simulink model "child"  (R2023a)
settings: Solver=FixedStepDiscrete  StartTime=0.0  StopTime=inf  RelTol=1e-3
undefined symbols (not defined in the file): child_1, dismiss
libraries: androidcommunicationlib x9, androidaudiovideolib x3, androidsensorlib x3, simulink x2, androiduilib x1
settings Model: SimulationMode=external  Creator=aashm  LastModifiedBy=agarw_crynhxp
settings OptimizationCC: BlockReduction=off  EnhancedBackFolding=on  PassReuseOutputArgsAs=Individual arguments  ZeroExternalMemoryAtStartup=off  ZeroInternalMemoryAtStartup=off  MaxStackSize=64  OptimizeBlockOrder=speed  DifferentSizesBufferReuse=on  OptimizationCustomize=off  EfficientTunableParamExpr=on
settings DebuggingCC: ParameterTunabilityLossMsg=error
settings HardwareCC: ProdBitPerPointer=32  ProdBitPerSizeT=32  ProdBitPerPtrDiffT=32  ProdLargestAtomicInteger=Long  ProdLargestAtomicFloat=Double  ProdWordSize=32  ProdHWDeviceType=ARM Compatible->ARM Cortex  UseEmbeddedCoderFeatures=off  UseSimulinkCoderFeatures=off
settings SFSimCC: MATLABDynamicMemAlloc=off
settings RTWCC: Description=Embedded Coder  SystemTargetFile=ert.tlc  HardwareBoard=Android Device  TLCOptions="-aInlineSetEventsForThisBaseRateFcn=TLC_FALSE -aSuppressMultiTaskScheduler=TLC_FALSE  -aRateBasedStepFcn=0"  TemplateMakefile=ert_default_tmf  RTWVerbose=off  Toolchain=Android SDK/NDK Tools
settings CodeAppCC: ForceParamTrailComments=on  IgnoreCustomStorageClasses=off  OperatorAnnotations=on  SimulinkDataObjDesc=on  SFDataObjDesc=on  InsertBlockDesc=on
settings ERTTargetCC: SupportNonInlinedSFcns=on

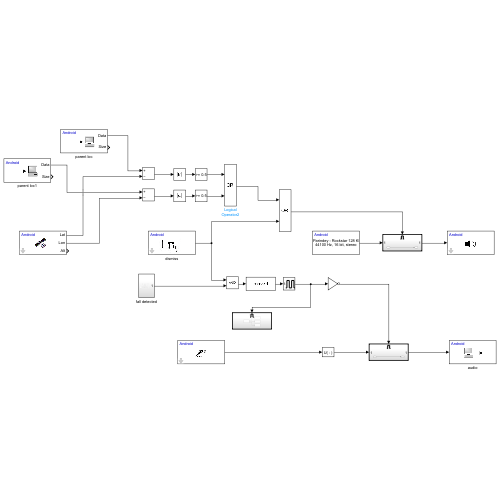
[thumbnail: Simulink's stored preview of the top-level diagram]
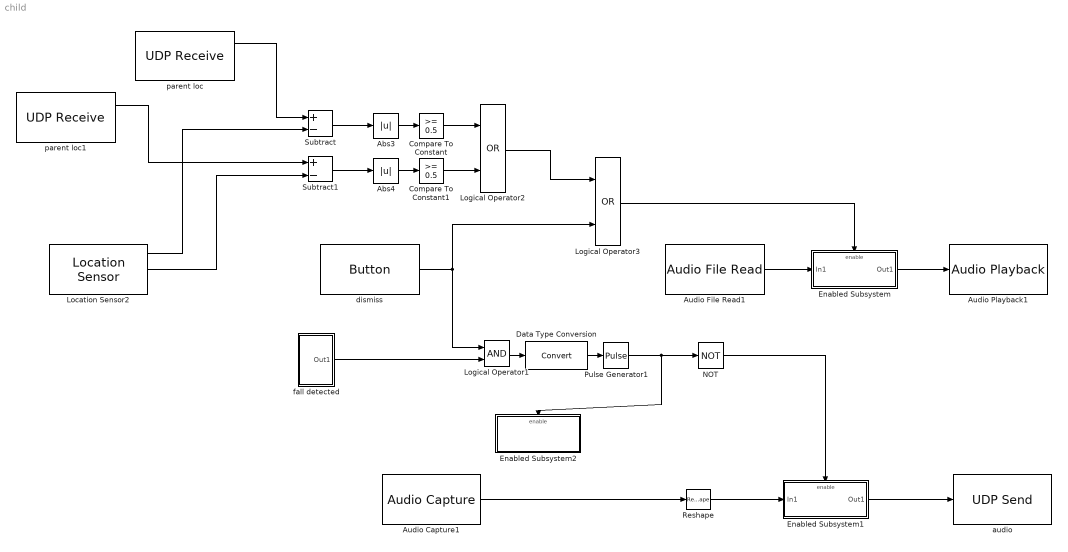
== system child ==
  Abs3 : Abs  OutDataTypeStr=int8  SaturateOnIntegerOverflow=off
  Abs4 : Abs  OutDataTypeStr=int8  SaturateOnIntegerOverflow=off
  Audio Capture1 : androidaudiovideolib/Audio Capture  SampleFreq=8000  FrameSize=80  SampleTime=0.01  SimulateUsing=Code generation  DeviceStr=0  QueueDuration=0  BlockPlatform=Android  AudioSamplingFreq=44100
  Audio File Read1 : androidaudiovideolib/Audio File Read  FileName=E:\agarw_crynhxp\Documents\Nadaan Parindey - Rockstar 128 Kbps.mp3  FrameSize=44100
  Audio Playback1 : androidaudiovideolib/Audio Playback  SampleFreq=44100  AudioSamplingFreq=44100  SampleTime=0.1  DeviceStr=0  QueueDuration=0  BlockPlatform=Android
  Compare To Constant : simulink/Logic and Bit Operations/Compare To Constant  relop=>=  const=0.5  OutDataTypeStr=boolean
  Compare To Constant1 : simulink/Logic and Bit Operations/Compare To Constant  relop=>=  const=0.5  OutDataTypeStr=boolean
  Data Type Conversion : DataTypeConversion  SaturateOnIntegerOverflow=off  RndMeth=Floor
  Enabled Subsystem : Subsystem  TreatAsAtomicUnit=on
  Enabled Subsystem1 : Subsystem  TreatAsAtomicUnit=on
  Enabled Subsystem2 : Subsystem  TreatAsAtomicUnit=on
  Location Sensor2 : androidsensorlib/Location Sensor  OutputVector=off  SampleTime=0.01  BlockPlatform=Android
  Logical Operator1 : Logic  AllPortsSameDT=off  OutDataTypeStr=fixdt(1,16)
  Logical Operator2 : Logic  Operator=OR  OutDataTypeStr=boolean
  Logical Operator3 : Logic  Operator=OR
  NOT : Logic  Operator=NOT  IconShape=distinctive  AllPortsSameDT=off
  Pulse Generator1 : DiscretePulseGenerator  PulseType=Time based  TimeSource=Use external signal  Period=100  PulseWidth=5
  Reshape : Reshape
  Subtract : Sum  Inputs=+-  OutDataTypeStr=int8
  Subtract1 : Sum  Inputs=+-  AccumDataTypeStr=int8  OutDataTypeStr=int8
  audio : androidcommunicationlib/UDP Send  remoteURL='10.7.20.4'  remotePort=30000  localURL='0.0.0.0'  localPortSource=Automatically determine  localPort=-1  sampletime=-1  blockPlatform=Android  separateLengthPort=0
  dismiss : androiduilib/Button  ButtonState=Pressed  ButtonId=child_1/dismiss  State=on  SampleTime=0.1  BlockPlatform=Android
  fall detected : Subsystem
  parent loc : androidcommunicationlib/UDP Receive  localURL='0.0.0.0'  localPort=40000  remoteURL='0.0.0.0'  remotePort=-1  recvBufferSize=8192  signalDatatype=uint8  dims=255  isVarSize=off  showBlockingTime=off  blockingTime=0  sampletime=0.01  blockPlatform=Android
  parent loc1 : androidcommunicationlib/UDP Receive  localURL='0.0.0.0'  localPort=45000  remoteURL='0.0.0.0'  remotePort=-1  recvBufferSize=8192  signalDatatype=uint8  dims=255  isVarSize=off  showBlockingTime=off  blockingTime=0  sampletime=0.01  blockPlatform=Android
  wires:
  dismiss/1 -> Logical Operator1/1, Logical Operator3/2
  Pulse Generator1/1 -> Enabled Subsystem2/Enable, NOT/1
  Enabled Subsystem1/1(Out1) -> audio/1
  Subtract/1 -> Abs3/1
  Compare To Constant/1 -> Logical Operator2/1
  Abs3/1 -> Compare To Constant/1
  Location Sensor2/1 -> Subtract/2
  Subtract1/1 -> Abs4/1
  Abs4/1 -> Compare To Constant1/1
  parent loc1/1 -> Subtract1/1
  Location Sensor2/2 -> Subtract1/2
  Compare To Constant1/1 -> Logical Operator2/2
  Audio Capture1/1 -> Reshape/1
  Reshape/1 -> Enabled Subsystem1/1(In1)
  Logical Operator2/1 -> Logical Operator3/1
  parent loc/1 -> Subtract/1
  Audio File Read1/1 -> Enabled Subsystem/1(In1)
  Logical Operator3/1 -> Enabled Subsystem/Enable
  Enabled Subsystem/1(Out1) -> Audio Playback1/1
  fall detected/1(Out1) -> Logical Operator1/2
  NOT/1 -> Enabled Subsystem1/Enable
  Logical Operator1/1 -> Data Type Conversion/1
  Data Type Conversion/1 -> Pulse Generator1/1

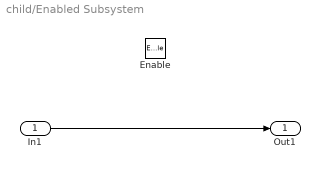
== system child/Enabled Subsystem ==
  In1 : Inport
  Enable : EnablePort
  Out1 : Outport
  wires:
  In1/1 -> Out1/1

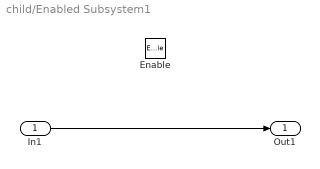
== system child/Enabled Subsystem1 ==
  In1 : Inport
  Enable : EnablePort
  Out1 : Outport
  wires:
  In1/1 -> Out1/1

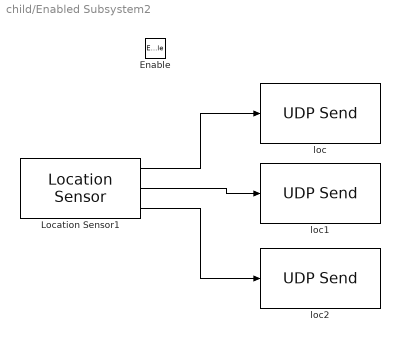
== system child/Enabled Subsystem2 ==
  Enable : EnablePort
  Location Sensor1 : androidsensorlib/Location Sensor  OutputVector=off  SampleTime=0.1  BlockPlatform=Android
  loc : androidcommunicationlib/UDP Send  remoteURL='10.7.20.4'  remotePort=50000  localURL='0.0.0.0'  localPortSource=Automatically determine  localPort=-1  sampletime=-1  blockPlatform=Android  separateLengthPort=0
  loc1 : androidcommunicationlib/UDP Send  remoteURL='10.7.20.4'  remotePort=55000  localURL='0.0.0.0'  localPortSource=Automatically determine  localPort=-1  sampletime=-1  blockPlatform=Android  separateLengthPort=0
  loc2 : androidcommunicationlib/UDP Send  remoteURL='10.7.20.4'  remotePort=60000  localURL='0.0.0.0'  localPortSource=Automatically determine  localPort=-1  sampletime=-1  blockPlatform=Android  separateLengthPort=0
  wires:
  Location Sensor1/2 -> loc1/1
  Location Sensor1/3 -> loc2/1
  Location Sensor1/1 -> loc/1

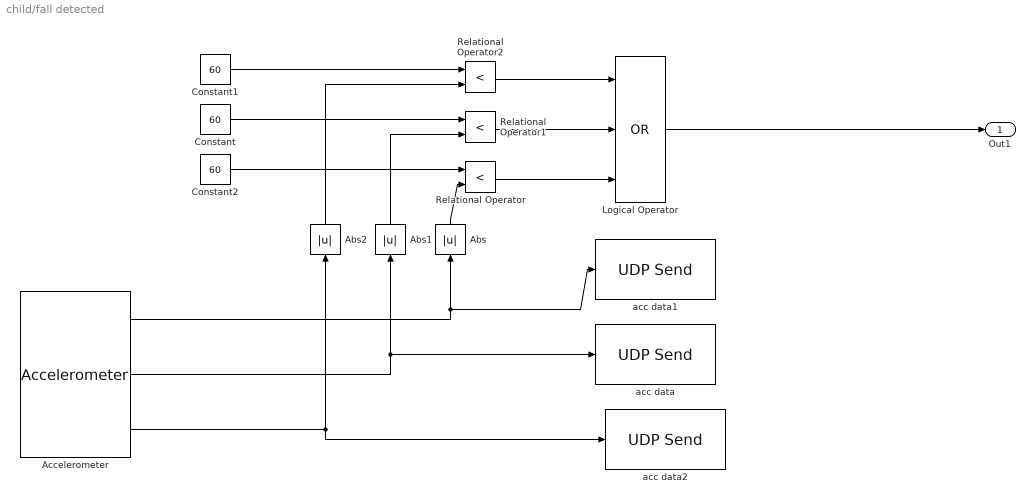
== system child/fall detected ==
  Abs : Abs  SaturateOnIntegerOverflow=off
  Abs1 : Abs  SaturateOnIntegerOverflow=off
  Abs2 : Abs  SaturateOnIntegerOverflow=off
  Accelerometer : androidsensorlib/Accelerometer  OutputVector=off  SampleTime=0.1  BlockPlatform=Android
  Constant : Constant  Value=60
  Constant1 : Constant  Value=60
  Constant2 : Constant  Value=60
  Logical Operator : Logic  Operator=OR  Inputs=3  AllPortsSameDT=off  OutDataTypeStr=fixdt(1,16)
  Relational Operator : RelationalOperator  Operator=<  OutDataTypeStr=fixdt(1,16)  RndMeth=Simplest  InputSameDT=off
  Relational Operator1 : RelationalOperator  Operator=<  OutDataTypeStr=fixdt(1,16)  RndMeth=Simplest  InputSameDT=off
  Relational Operator2 : RelationalOperator  Operator=<  OutDataTypeStr=fixdt(1,16)  RndMeth=Simplest  InputSameDT=off
  acc data : androidcommunicationlib/UDP Send  remoteURL='10.7.20.4'  remotePort=15000  localURL='0.0.0.0'  localPortSource=Automatically determine  localPort=-1  sampletime=-1  blockPlatform=Android  separateLengthPort=0
  acc data1 : androidcommunicationlib/UDP Send  remoteURL='10.7.20.4'  remotePort=25000  localURL='0.0.0.0'  localPortSource=Automatically determine  localPort=-1  sampletime=-1  blockPlatform=Android  separateLengthPort=0
  acc data2 : androidcommunicationlib/UDP Send  remoteURL='10.7.20.4'  remotePort=20000  localURL='0.0.0.0'  localPortSource=Automatically determine  localPort=-1  sampletime=-1  blockPlatform=Android  separateLengthPort=0
  Out1 : Outport
  wires:
  Constant/1 -> Relational Operator1/1
  Accelerometer/3 -> Abs2/1, acc data2/1
  Accelerometer/1 -> Abs/1, acc data1/1
  Abs2/1 -> Relational Operator2/2
  Relational Operator1/1 -> Logical Operator/2
  Relational Operator2/1 -> Logical Operator/1
  Constant2/1 -> Relational Operator/1
  Relational Operator/1 -> Logical Operator/3
  Abs/1 -> Relational Operator/2
  Abs1/1 -> Relational Operator1/2
  Accelerometer/2 -> Abs1/1, acc data/1
  Constant1/1 -> Relational Operator2/1
  Logical Operator/1 -> Out1/1
